simulink model "ComparacionPIDconPI"  (R2023b)
settings: Solver=VariableStepAuto  StartTime=0.0  StopTime=10.0  RelTol=1e-3
settings Model: Creator=Angel Garcia  LastModifiedBy=Angel Garcia

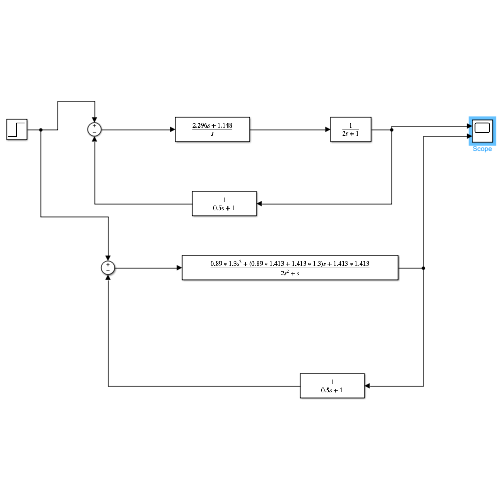
[thumbnail: Simulink's stored preview of the top-level diagram]
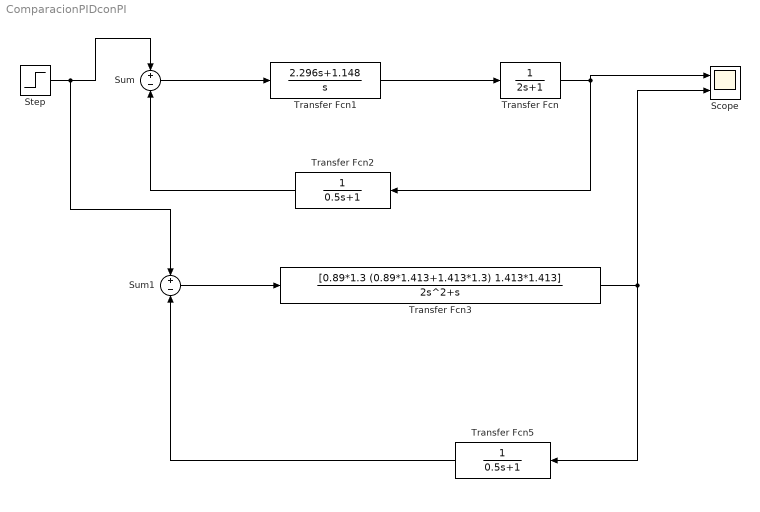
== system ComparacionPIDconPI ==
  Scope : Scope  NumInputPorts=2
  Step : Step  SampleTime=0
  Sum : Sum  Inputs=+-
  Sum1 : Sum  Inputs=+-
  Transfer Fcn : TransferFcn  Denominator=[2 1]
  Transfer Fcn1 : TransferFcn  Numerator=[2.296 1.148]  Denominator=[1 0]
  Transfer Fcn2 : TransferFcn  Denominator=[0.5 1]
  Transfer Fcn3 : TransferFcn  Numerator=[0.89*1.3 (0.89*1.413+1.413*1.3) 1.413*1.413]  Denominator=[2 1 0]  AbsoluteTolerance=Auto
  Transfer Fcn5 : TransferFcn  Denominator=[0.5 1]
  wires:
  Sum/1 -> Transfer Fcn1/1
  Transfer Fcn1/1 -> Transfer Fcn/1
  Transfer Fcn/1 -> Scope/1, Transfer Fcn2/1
  Transfer Fcn2/1 -> Sum/2
  Transfer Fcn3/1 -> Scope/2, Transfer Fcn5/1
  Sum1/1 -> Transfer Fcn3/1
  Transfer Fcn5/1 -> Sum1/2
  Step/1 -> Sum1/1, Sum/1
